simulink library "SUB_ECU_L4_MABX"  (R2018a)
settings: Solver=VariableStepAuto  StartTime=0.0  StopTime=10.0  RelTol=1e-3
libraries: EmE_MBD_Blockset x76, simulink x14, SUB_L4_Task_10000ms x1, SUB_L4_Task_1000ms x1, SUB_L4_Task_100ms x1, SUB_L4_Task_10ms_SUB_APTC x1, PTC_MBDS_LIB x1, SUB_L4_Task_10ms_SUB_BRKPEDARB x1, SUB_L4_Task_10ms_SUB_FAULT_MANAGER x1, SUB_L4_Task_10ms_SUB_STATE_CONTROL x1, SUB_L4_Task_10ms_SUB_STEERCTRL x1, simulink_need_slupdate x1
(part 2 of 2)

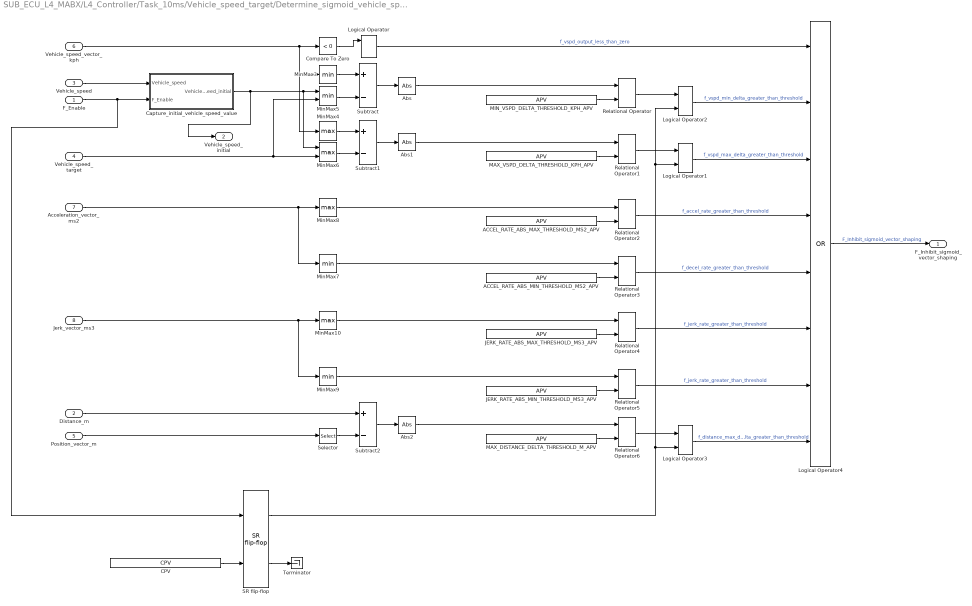
== system SUB_ECU_L4_MABX/L4_Controller/Task_10ms/Vehicle_speed_target/Determine_sigmoid_vehicle_speed_profile/Determine_inhibit_sigmoid_vehicle_speed_profile ==
  F_Enable : Inport
  Distance_m : Inport  Port=2
  Vehicle_speed : Inport  Port=3
  Vehicle_speed_target : Inport  Port=4
  Position_vector_m : Inport  Port=5
  Vehicle_speed_vector_kph : Inport  Port=6
  Acceleration_vector_ms2 : Inport  Port=7
  Jerk_vector_ms3 : Inport  Port=8
  ACCEL_RATE_ABS_MAX_THRESHOLD_MS2_APV : EmE_MBD_Blockset/Sources/APV  conval=5
      settings: SourceProductName=PACCAR EmE MBD Blockset
  ACCEL_RATE_ABS_MIN_THRESHOLD_MS2_APV : EmE_MBD_Blockset/Sources/APV  conval=-5
      settings: SourceProductName=PACCAR EmE MBD Blockset
  Abs : EmE_MBD_Blockset/Math Operators/Abs
      settings: SourceProductName=PACCAR EmE MBD Blockset
  Abs1 : EmE_MBD_Blockset/Math Operators/Abs
      settings: SourceProductName=PACCAR EmE MBD Blockset
  Abs2 : EmE_MBD_Blockset/Math Operators/Abs
      settings: SourceProductName=PACCAR EmE MBD Blockset
  CPV : EmE_MBD_Blockset/Sources/CPV  conval=false
      settings: SourceProductName=PACCAR EmE MBD Blockset
  Capture_initial_vehicle_speed_value : Subsystem
  Compare To Zero : simulink/Logic and Bit Operations/Compare To Zero  relop=<  OutDataTypeStr=boolean
  JERK_RATE_ABS_MAX_THRESHOLD_MS3_APV : EmE_MBD_Blockset/Sources/APV  conval=5
      settings: SourceProductName=PACCAR EmE MBD Blockset
  JERK_RATE_ABS_MIN_THRESHOLD_MS3_APV : EmE_MBD_Blockset/Sources/APV  conval=-5
      settings: SourceProductName=PACCAR EmE MBD Blockset
  Logical Operator : EmE_MBD_Blockset/Logic and Bit Operations/Logical Operator  Operator=OR  Inputs=1
      settings: SourceProductName=PACCAR EmE MBD Blockset
  Logical Operator1 : EmE_MBD_Blockset/Logic and Bit Operations/Logical Operator  Operator=AND  Inputs=2
      settings: SourceProductName=PACCAR EmE MBD Blockset
  Logical Operator2 : EmE_MBD_Blockset/Logic and Bit Operations/Logical Operator  Operator=AND  Inputs=2
      settings: SourceProductName=PACCAR EmE MBD Blockset
  Logical Operator3 : EmE_MBD_Blockset/Logic and Bit Operations/Logical Operator  Operator=AND  Inputs=2
      settings: SourceProductName=PACCAR EmE MBD Blockset
  Logical Operator4 : Logic  Operator=OR  Inputs=8  AllPortsSameDT=off  OutDataTypeStr=boolean
  MAX_DISTANCE_DELTA_THRESHOLD_M_APV : EmE_MBD_Blockset/Sources/APV  conval=0.5
      settings: SourceProductName=PACCAR EmE MBD Blockset
  MAX_VSPD_DELTA_THRESHOLD_KPH_APV : EmE_MBD_Blockset/Sources/APV  conval=5
      settings: SourceProductName=PACCAR EmE MBD Blockset
  MIN_VSPD_DELTA_THRESHOLD_KPH_APV : EmE_MBD_Blockset/Sources/APV  conval=5
      settings: SourceProductName=PACCAR EmE MBD Blockset
  MinMax10 : MinMax  Function=max  InputSameDT=on
  MinMax3 : MinMax  InputSameDT=on
  MinMax4 : MinMax  Function=max  InputSameDT=on
  MinMax5 : MinMax  Inputs=2  InputSameDT=on
  MinMax6 : MinMax  Function=max  Inputs=2  InputSameDT=on
  MinMax7 : MinMax  InputSameDT=on
  MinMax8 : MinMax  Function=max  InputSameDT=on
  MinMax9 : MinMax  InputSameDT=on
  Relational Operator{,1..2,4,6} (5 alike) : EmE_MBD_Blockset/Logic and Bit Operations/Relational Operator  func=>
      settings: SourceProductName=PACCAR EmE MBD Blockset
  Relational Operator3 : EmE_MBD_Blockset/Logic and Bit Operations/Relational Operator  func=<
      settings: SourceProductName=PACCAR EmE MBD Blockset
  Relational Operator5 : EmE_MBD_Blockset/Logic and Bit Operations/Relational Operator  func=<
      settings: SourceProductName=PACCAR EmE MBD Blockset
  SR flip-flop : EmE_MBD_Blockset/Logic and Bit Operations/SR flip-flop
      settings: SourceProductName=PACCAR EmE MBD Blockset
  Selector : Selector  InputPortWidth=33  IndexOptions=Index vector (dialog)  Indices=33  OutputSizes=1
  Subtract : Sum  Inputs=+-  InputSameDT=on
  Subtract1 : Sum  Inputs=+-  InputSameDT=on
  Subtract2 : Sum  Inputs=+-  InputSameDT=on
  Terminator : Terminator
  F_Inhibit_sigmoid_vector_shaping : Outport  LibraryBlock=EmE_MBD_Blockset/Sinks/Out  OutputWhenDisabled=reset
  Vehicle_speed_initial : Outport  Port=2
  wires:
  Relational Operator6/1 -> Logical Operator3/1
  Position_vector_m/1 -> Selector/1
  Selector/1 -> Subtract2/2
  Logical Operator3/1 -> Logical Operator4/8  "f_distance_max_delta_greater_than_threshold"
  Distance_m/1 -> Subtract2/1
  Subtract2/1 -> Abs2/1
  Abs2/1 -> Relational Operator6/1
  MAX_DISTANCE_DELTA_THRESHOLD_M_APV/1 -> Relational Operator6/2
  Vehicle_speed/1 -> Capture_initial_vehicle_speed_value/1(Vehicle_speed)
  Capture_initial_vehicle_speed_value/1(Vehicle_speed_initial) -> MinMax5/1, MinMax6/1, Vehicle_speed_initial/1
  Vehicle_speed_target/1 -> MinMax6/2, MinMax5/2
  MinMax6/1 -> Subtract1/2
  MinMax5/1 -> Subtract/2
  Subtract/1 -> Abs/1
  Subtract1/1 -> Abs1/1
  Relational Operator1/1 -> Logical Operator1/1
  MAX_VSPD_DELTA_THRESHOLD_KPH_APV/1 -> Relational Operator1/2
  Logical Operator2/1 -> Logical Operator4/2  "f_vspd_min_delta_greater_than_threshold"
  MinMax9/1 -> Relational Operator5/1
  JERK_RATE_ABS_MIN_THRESHOLD_MS3_APV/1 -> Relational Operator5/2
  Logical Operator/1 -> Logical Operator4/1  "f_vspd_output_less_than_zero"
  MinMax4/1 -> Subtract1/1
  MIN_VSPD_DELTA_THRESHOLD_KPH_APV/1 -> Relational Operator/2
  Jerk_vector_ms3/1 -> MinMax10/1, MinMax9/1
  Abs1/1 -> Relational Operator1/1
  Abs/1 -> Relational Operator/1
  Logical Operator1/1 -> Logical Operator4/3  "f_vspd_max_delta_greater_than_threshold"
  Relational Operator5/1 -> Logical Operator4/7  "f_jerk_rate_greater_than_threshold"
  MinMax10/1 -> Relational Operator4/1
  ACCEL_RATE_ABS_MAX_THRESHOLD_MS2_APV/1 -> Relational Operator2/2
  MinMax8/1 -> Relational Operator2/1
  Relational Operator/1 -> Logical Operator2/1
  JERK_RATE_ABS_MAX_THRESHOLD_MS3_APV/1 -> Relational Operator4/2
  Acceleration_vector_ms2/1 -> MinMax8/1, MinMax7/1
  Vehicle_speed_vector_kph/1 -> Compare To Zero/1, MinMax3/1, MinMax4/1
  Relational Operator2/1 -> Logical Operator4/4  "f_accel_rate_greater_than_threshold"
  Relational Operator3/1 -> Logical Operator4/5  "f_decel_rate_greater_than_threshold"
  MinMax3/1 -> Subtract/1
  SR flip-flop/1 -> Logical Operator2/2, Logical Operator1/2, Logical Operator3/2
  MinMax7/1 -> Relational Operator3/1
  SR flip-flop/2 -> Terminator/1
  Relational Operator4/1 -> Logical Operator4/6  "f_jerk_rate_greater_than_threshold"
  CPV/1 -> SR flip-flop/2
  Logical Operator4/1 -> F_Inhibit_sigmoid_vector_shaping/1  "F_Inhibit_sigmoid_vector_shaping"
  ACCEL_RATE_ABS_MIN_THRESHOLD_MS2_APV/1 -> Relational Operator3/2
  F_Enable/1 -> Capture_initial_vehicle_speed_value/2(F_Enable), SR flip-flop/1
  Compare To Zero/1 -> Logical Operator/1

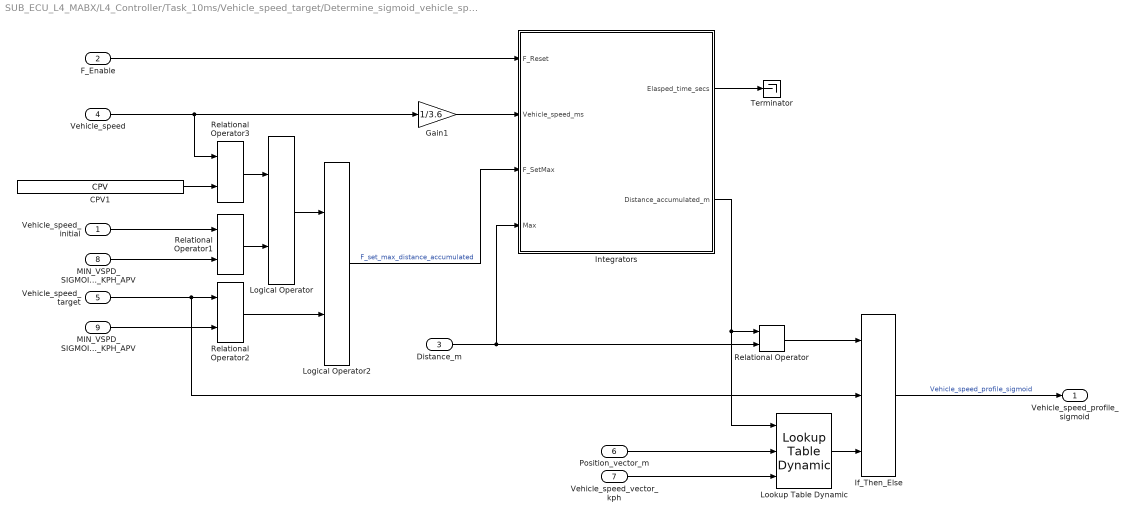
== system SUB_ECU_L4_MABX/L4_Controller/Task_10ms/Vehicle_speed_target/Determine_sigmoid_vehicle_speed_profile/Select_vehicle_speed_target_value ==
  Vehicle_speed_initial : Inport
  F_Enable : Inport  Port=2
  Distance_m : Inport  Port=3
  Vehicle_speed : Inport  Port=4
  Vehicle_speed_target : Inport  Port=5
  Position_vector_m : Inport  Port=6
  Vehicle_speed_vector_kph : Inport  Port=7
  MIN_VSPD_SIGMOID_INITIAL_KPH_APV : Inport  Port=8
  MIN_VSPD_SIGMOID_FINAL_KPH_APV : Inport  Port=9
  CPV1 : EmE_MBD_Blockset/Sources/CPV  conval=0.1
      settings: SourceProductName=PACCAR EmE MBD Blockset
  Gain1 : Gain  Gain=1/3.6
  If_Then_Else : EmE_MBD_Blockset/Signal Routing/If_Then_Else
      settings: SourceProductName=PACCAR EmE MBD Blockset
  Integrators : Subsystem
  Logical Operator : EmE_MBD_Blockset/Logic and Bit Operations/Logical Operator  Operator=OR  Inputs=2
      settings: SourceProductName=PACCAR EmE MBD Blockset
  Logical Operator2 : EmE_MBD_Blockset/Logic and Bit Operations/Logical Operator  Operator=AND  Inputs=2
      settings: SourceProductName=PACCAR EmE MBD Blockset
  Lookup Table Dynamic : simulink/Lookup Tables/Lookup Table Dynamic  LookUpMeth=Interpolation-Use End Values  OutDataType=fixdt('double')  OutScaling=[]  OutputDataTypeScalingMode=Specify via dialog  OutDataTypeStr=double  DoSatur=off
      settings: SourceProductName=Simulink
  Relational Operator : EmE_MBD_Blockset/Logic and Bit Operations/Relational Operator  func===
      settings: SourceProductName=PACCAR EmE MBD Blockset
  Relational Operator1 : EmE_MBD_Blockset/Logic and Bit Operations/Relational Operator  func=<
      settings: SourceProductName=PACCAR EmE MBD Blockset
  Relational Operator2 : EmE_MBD_Blockset/Logic and Bit Operations/Relational Operator  func=<
      settings: SourceProductName=PACCAR EmE MBD Blockset
  Relational Operator3 : EmE_MBD_Blockset/Logic and Bit Operations/Relational Operator  func=<
      settings: SourceProductName=PACCAR EmE MBD Blockset
  Terminator : Terminator
  Vehicle_speed_profile_sigmoid : Outport
  wires:
  Logical Operator2/1 -> Integrators/3(F_SetMax)  "F_set_max_distance_accumulated"
  CPV1/1 -> Relational Operator3/2
  Relational Operator1/1 -> Logical Operator/2
  Logical Operator/1 -> Logical Operator2/1
  Relational Operator3/1 -> Logical Operator/1
  Relational Operator/1 -> If_Then_Else/1
  Gain1/1 -> Integrators/2(Vehicle_speed_ms)
  Integrators/2(Distance_accumulated_m) -> Relational Operator/1, Lookup Table Dynamic/1
  MIN_VSPD_SIGMOID_FINAL_KPH_APV/1 -> Relational Operator2/2
  MIN_VSPD_SIGMOID_INITIAL_KPH_APV/1 -> Relational Operator1/2
  Relational Operator2/1 -> Logical Operator2/2
  Vehicle_speed_initial/1 -> Relational Operator1/1
  F_Enable/1 -> Integrators/1(F_Reset)
  Lookup Table Dynamic/1 -> If_Then_Else/3
  Vehicle_speed_vector_kph/1 -> Lookup Table Dynamic/3
  Integrators/1(Elasped_time_secs) -> Terminator/1
  Position_vector_m/1 -> Lookup Table Dynamic/2
  Vehicle_speed/1 -> Gain1/1, Relational Operator3/1
  Distance_m/1 -> Integrators/4(Max), Relational Operator/2
  If_Then_Else/1 -> Vehicle_speed_profile_sigmoid/1  "Vehicle_speed_profile_sigmoid"
  Vehicle_speed_target/1 -> Relational Operator2/1, If_Then_Else/2

== system SUB_ECU_L4_MABX/L4_Controller/Task_10ms/Vehicle_speed_target/Determine_sigmoid_vehicle_speed_profile/Determine_inhibit_sigmoid_vehicle_speed_profile/Capture_initial_vehicle_speed_value ==
  Vehicle_speed : Inport
  F_Enable : Inport  Port=2
  If_Then_Else : EmE_MBD_Blockset/Signal Routing/If_Then_Else
      settings: SourceProductName=PACCAR EmE MBD Blockset
  Unit_Delay : UnitDelay  SampleTime=-1
      settings: AttributesFormatString=IC: %<vinit>
  Vehicle_speed_initial : Outport
  wires:
  Vehicle_speed/1 -> If_Then_Else/2
  Unit_Delay/1 -> If_Then_Else/3
  F_Enable/1 -> If_Then_Else/1
  If_Then_Else/1 -> Vehicle_speed_initial/1, Unit_Delay/1  "Vehicle_speed_initial"

== system SUB_ECU_L4_MABX/L4_Controller/Task_10ms/Vehicle_speed_target/Determine_sigmoid_vehicle_speed_profile/Select_vehicle_speed_target_value/Integrators ==
  F_Reset : Inport
  Vehicle_speed_ms : Inport  Port=2
  F_SetMax : Inport  Port=3
  Max : Inport  Port=4
  CPV : EmE_MBD_Blockset/Sources/CPV  conval=1
      settings: SourceProductName=PACCAR EmE MBD Blockset
  CPV1 : EmE_MBD_Blockset/Sources/CPV  conval=1
      settings: SourceProductName=PACCAR EmE MBD Blockset
  CPV2 : EmE_MBD_Blockset/Sources/CPV  conval=1
      settings: SourceProductName=PACCAR EmE MBD Blockset
  CalculateDistance : Subsystem
  Discrete-Time Integrator : EmE_MBD_Blockset/Discrete/Discrete-Time Integrator  integrator_method_sel=Backward Euler
      settings: AttributesFormatString=%<integrator_method_sel>  SourceProductName=PACCAR EmE MBD Blockset
  dT : EmE_MBD_Blockset/Sources/dT
      settings: SourceProductName=PACCAR EmE MBD Blockset
  dT1 : EmE_MBD_Blockset/Sources/dT
      settings: SourceProductName=PACCAR EmE MBD Blockset
  Elasped_time_secs : Outport
  Distance_accumulated_m : Outport  Port=2
  wires:
  F_SetMax/1 -> CalculateDistance/5(F_SetMax)
  Max/1 -> CalculateDistance/6(Max)
  CPV2/1 -> Discrete-Time Integrator/2
  CPV1/1 -> CalculateDistance/3(K)
  dT1/1 -> CalculateDistance/4(dT)
  Discrete-Time Integrator/1 -> Elasped_time_secs/1  "Elasped_time_secs"
  F_Reset/1 -> Discrete-Time Integrator/1, CalculateDistance/1(F_Reset)
  Vehicle_speed_ms/1 -> CalculateDistance/2(U)
  CPV/1 -> Discrete-Time Integrator/3
  CalculateDistance/1(Y) -> Distance_accumulated_m/1  "Distance_accumulated_m"
  dT/1 -> Discrete-Time Integrator/4

== system SUB_ECU_L4_MABX/L4_Controller/Task_10ms/Vehicle_speed_target/Determine_sigmoid_vehicle_speed_profile/Select_vehicle_speed_target_value/Integrators/CalculateDistance ==
  F_Reset : Inport
  U : Inport  Port=2
  K : Inport  Port=3
  dT : Inport  Port=4
  F_SetMax : Inport  Port=5
  Max : Inport  Port=6
  Add : Sum  InputSameDT=on
  CPV : EmE_MBD_Blockset/Sources/CPV  conval=0
      settings: SourceProductName=PACCAR EmE MBD Blockset
  If_Then_Else : EmE_MBD_Blockset/Signal Routing/If_Then_Else
      settings: SourceProductName=PACCAR EmE MBD Blockset
  MinMax : MinMax  Inputs=2  InputSameDT=on
  Product1 : Product  Inputs=3  InputSameDT=on
  Unit Delay Resettable External IC1 : simulink_need_slupdate/Unit Delay Resettable External IC  tsamp=-1
      settings: SourceProductName=Simulink  SourceProductBaseCode=SL
  Y : Outport  OutputWhenDisabled=reset  InitialOutput=0
  wires:
  F_Reset/1 -> Unit Delay Resettable External IC1/2
  Product1/1 -> Add/2
  Add/1 -> MinMax/2
  CPV/1 -> Unit Delay Resettable External IC1/3
  Unit Delay Resettable External IC1/1 -> Add/1
  If_Then_Else/1 -> Y/1, Unit Delay Resettable External IC1/1
  MinMax/1 -> If_Then_Else/3
  F_SetMax/1 -> If_Then_Else/1
  Max/1 -> If_Then_Else/2, MinMax/1
  dT/1 -> Product1/3
  K/1 -> Product1/1
  U/1 -> Product1/2

== stateflow chart SUB_ECU_L4_MABX/L4_Controller/Task_10ms/Vehicle_speed_target/Determine_sigmoid_vehicle_speed_profile/TwentyPointVectorCalculation ==
  (default) -> (junction 85)
  (junction 85) -> (junction 86) [order 1] : [Enable]
  (junction 85) -> (junction 87) [order 2]
  (junction 86) -> (junction 21) : {TimeVector(1) = TimeVectorRaw(1);
      | JerkVector(1) = JerkVectorRaw(1);
      | AccelerationVector(1) = AccelerationVectorRaw(1);
      | VelocityVector(1) = VelocityVectorRaw(1);
      | PositionVector(1) = PositionVectorRaw(1);
      |
      | TimeIncrement = (TimeVectorRaw(2) - TimeVectorRaw(1)) / 10;
      | i = 2;}
  (junction 21) -> (junction 19) [order 1] : [i <= 10]
  (junction 19) -> (junction 22) : {TimeVector(i) = TimeVector(i-1) + TimeIncrement;
      | DeltaTime = TimeVector(i) - TimeVectorRaw(1);
      | JerkVector(i) = JerkVectorRaw(1);
      | AccelerationVector(i) = AccelerationVectorRaw(1) + JerkVectorRaw(1) * DeltaTime;
      | VelocityVector(i) = VelocityVectorRaw(1) + AccelerationVectorRaw(1) * DeltaTime + 0.5 * JerkVectorRaw(1) * DeltaTime^2;
      | PositionVector(i) = PositionVectorRaw(1) + VelocityVectorRaw(1) * DeltaTime + 0.5 * AccelerationVectorRaw(1) * DeltaTime^2 + (JerkVectorRaw(1) / 6) * DeltaTime^3;
      | PositionVector(i) = max(PositionVector(i-1) + 0.0001, PositionVector(i));}
  (junction 22) -> (junction 21) : {i = i + 1;}
  (junction 21) -> (junction 129) [order 2] : {TimeVector(11) = TimeVectorRaw(2);
      | JerkVector(11) = JerkVectorRaw(2);
      | AccelerationVector(11) = AccelerationVectorRaw(2);
      | VelocityVector(11) = VelocityVectorRaw(2);
      | PositionVector(11) = max(PositionVector(10) + 0.0001, PositionVectorRaw(2));
      |
      | TimeVector(12) = TimeVectorRaw(3);
      | JerkVector(12) = JerkVectorRaw(3);
      | AccelerationVector(12) = AccelerationVectorRaw(3);
      | VelocityVector(12) = VelocityVectorRaw(3);
      | PositionVector(12) = max(PositionVector(11) + 0.0001, PositionVectorRaw(3));
      |
      | TimeIncrement = (TimeVectorRaw(4) - TimeVectorRaw(3)) / 10;
      | i = 13;}
  (junction 129) -> (junction 128) [order 1] : [i <= 21]
  (junction 128) -> (junction 130) : {TimeVector(i) = TimeVector(i-1) + TimeIncrement;
      | DeltaTime = TimeVector(i) - TimeVectorRaw(3);
      | JerkVector(i) = JerkVectorRaw(3);
      | AccelerationVector(i) = AccelerationVectorRaw(3) + JerkVectorRaw(3) * DeltaTime;
      | VelocityVector(i) = VelocityVectorRaw(3) + AccelerationVectorRaw(3) * DeltaTime + 0.5 * JerkVectorRaw(3) * DeltaTime^2;
      | PositionVector(i) = PositionVectorRaw(3) + VelocityVectorRaw(3) * DeltaTime + 0.5 * AccelerationVectorRaw(3) * DeltaTime^2 + (JerkVectorRaw(3) / 6) * DeltaTime^3;
      | PositionVector(i) = max(PositionVector(i-1) + 0.0001, PositionVector(i));}
  (junction 130) -> (junction 129) : {i = i + 1;}
  (junction 129) -> (junction 109) [order 2] : {TimeVector(22) = TimeVectorRaw(4);
      | JerkVector(22) = JerkVectorRaw(4);
      | AccelerationVector(22) = AccelerationVectorRaw(4);
      | VelocityVector(22) = VelocityVectorRaw(4);
      | PositionVector(22) = max(PositionVector(21) + 0.0001, PositionVectorRaw(4));
      |
      | TimeVector(23) = TimeVectorRaw(5);
      | JerkVector(23) = JerkVectorRaw(5);
      | AccelerationVector(23) = AccelerationVectorRaw(5);
      | VelocityVector(23) = VelocityVectorRaw(5);
      | PositionVector(23) = max(PositionVector(22) + 0.0001, PositionVectorRaw(5));
      |
      | TimeIncrement = (TimeVectorRaw(6) - TimeVectorRaw(5)) / 10;
      | i = 24;}
  (junction 109) -> (junction 107) [order 1] : [i <= 32]
  (junction 107) -> (junction 108) : {TimeVector(i) = TimeVector(i-1) + TimeIncrement;
      | DeltaTime = TimeVector(i) - TimeVectorRaw(5);
      | JerkVector(i) = JerkVectorRaw(5);
      | AccelerationVector(i) = AccelerationVectorRaw(5) + JerkVectorRaw(5) * DeltaTime;
      | VelocityVector(i) = VelocityVectorRaw(5) + AccelerationVectorRaw(5) * DeltaTime + 0.5 * JerkVectorRaw(5) * DeltaTime^2;
      | PositionVector(i) = PositionVectorRaw(5) + VelocityVectorRaw(5) * DeltaTime + 0.5 * AccelerationVectorRaw(5) * DeltaTime^2 + (JerkVectorRaw(5) / 6) * DeltaTime^3;
      | PositionVector(i) = max(PositionVector(i-1) + 0.0001, PositionVector(i));}
  (junction 108) -> (junction 109) : {i = i + 1;}
  (junction 109) -> (junction 23) [order 2] : {TimeVector(33) = TimeVectorRaw(6);
      | JerkVector(33) = JerkVectorRaw(6);
      | AccelerationVector(33) = AccelerationVectorRaw(6);
      | VelocityVector(33) = VelocityVectorRaw(6);
      | PositionVector(33) = max(PositionVector(32) + 0.0001, PositionVectorRaw(6));}
  (junction 23) -> (junction 87)
  (junction 87) -> (junction 92)
  data: TimeVector output size=33 =[0:0.001:0.032]'; PositionVector output size=33 =[0:0.001:0.032]'; VelocityVector output size=33 =zeros(33,1); AccelerationVector output size=33 =zeros(33,1); JerkVector output size=33 =zeros(33,1); Enable input; PositionFinal input; TimeVectorRaw input; PositionVectorRaw input; VelocityVectorRaw input; AccelerationVectorRaw input; JerkVectorRaw input; i local uint8; DeltaTime local double; TimeIncrement local double

== stateflow chart SUB_ECU_L4_MABX/L4_Controller/Task_10ms/Vehicle_speed_target/Determine_sigmoid_vehicle_speed_profile/VehicleSpeedSetpointDynamicCalculation ==
  state CalculateAcceleration34 [function]
    (default) -> (junction 180) : {num = 2 * (AccelerationInitialLimited *  AccelerationFinalLimited ...
        |     - AccelerationInitialLimited * Jerk56 * TimeFinal ...
        |     + Jerk56 * (VelocityFinalLimited - VelocityInitialLimited)) ...
        |     - AccelerationInitialLimited^2 - AccelerationFinalLimited^2;
        |
        | den = 2 * ((VelocityFinalLimited - VelocityInitialLimited) ...
        |     - AccelerationFinalLimited * TimeFinal) ...
        |     + Jerk56 * TimeFinal^2;
        |
        | Jerk12 = sign(Jerk12) * max(abs(Jerk12), abs(num / den) + 0.001);
        | Jerk12 = max(-10,min(10,Jerk12));
        |
        | Calculate_abc}
    (junction 180) -> (junction 181) [order 1] : [abs(a) < 0.01 ]
    (junction 180) -> (junction 205) [order 2]
    (junction 181) -> (junction 183) : {Jerk12 = Jerk56;
        | Calculate_abc
        | Acceleration34 = - c / b;
        | AlternateMethod = false;}
    (junction 205) -> (junction 291) [order 1] : [b^2 <= 4 * a * c]
    (junction 205) -> (junction 288) [order 2] : {Acceleration34 = (- b + (b^2 - 4 * a * c)^0.5) / (2 * a);
        | AlternateMethod = false;}
    (junction 291) -> (junction 290) : {CalculateAlternate_abc
        | Acceleration34 = - b / (2 * a);
        | AlternateMethod = true;}
    (junction 290) -> (junction 288)
    (junction 183) -> (junction 290)
    (junction 288) -> (junction 189)
  state Calculate_abc [function]
    (default) -> (junction 164) : {a = Jerk56 - Jerk12;
        | b = 2 * (AccelerationFinalLimited * Jerk12 - AccelerationInitialLimited * Jerk56 - Jerk12 * Jerk56 * TimeFinal);
        | c = 2 * Jerk12 * Jerk56 * (VelocityFinalLimited - VelocityInitialLimited) + Jerk56 * AccelerationInitialLimited^2 - Jerk12 * AccelerationFinalLimited^2;}
  state CalculateAlternate_abc [function]
    (default) -> (junction 287) : {a = 1;
        | b = 2 * (Jerk56 * (TimeFinal - 0.005) - AccelerationFinalLimited);
        | c = 2 * Jerk56 * (VelocityInitialLimited - VelocityFinalLimited) + AccelerationFinalLimited^2;}
  (default) -> (junction 85)
  (junction 85) -> (junction 86) [order 1] : [Enable]
  (junction 85) -> (junction 87) [order 2]
  (junction 86) -> (junction 236) : {PositionFinalLimited = max(0.001,PositionFinal);  % limit minimum distance so that values in PositionVectorRaw are in increasing order
      |
      | VelocityInitialLimited = max(0.1,VelocityInitial);  % limit to make sure FinalTime calculation does not divide by zero
      | VelocityFinalLimited = max(0.1,VelocityFinal);  % limit to make sure FinalTime calculation does not divide by zero
      |
      | TimeFinal = 2 * PositionFinalLimited / (VelocityInitialLimited + VelocityFinalLimited);  % first approximation for total time
      | TimeFinal = max(0.007, TimeFinal);  % limit to make sure values in JerkVectorRaw are in increasing order and divide by zero protection
      |  AccelerationAverage = (VelocityFinalLimited - VelocityInitialLimited) / TimeFinal;   % acceleration with straight line velocity change
      | TimeFinal = 2 * TimeFinal;  % increase initial estimate two times to make sure solution is within search range
      | }
  (junction 236) -> (junction 237) [order 1] : [VelocityFinalLimited > VelocityInitialLimited]
  (junction 236) -> (junction 38) [order 2] : {% deceleration sigmoid limits
      | AccelerationInitialLimited = max(AccelerationAverage, min(0, AccelerationInitial));
      | AccelerationFinalLimited = max(AccelerationAverage, min(0, AccelerationFinal));}
  (junction 237) -> (junction 239) : {% acceleration sigmoid limits
      | AccelerationInitialLimited = max(0, min(AccelerationAverage, AccelerationInitial));
      | AccelerationFinalLimited = max(0, min(AccelerationAverage, AccelerationFinal));}
  (junction 239) -> (junction 38)
  (junction 38) -> (junction 21) : {DeltaTimeFinal = TimeFinal;  % initialize DeltaTimeFinal term for binary search
      | i = 1;}
  (junction 21) -> (junction 19) [order 1] : % TimeFinal
      | % Binary Search
      |
      | [i <= 15]
  (junction 19) -> (junction 115) : {JerkFinalMinimum = 2 * (VelocityInitialLimited - VelocityFinalLimited + AccelerationFinalLimited * TimeFinal) / TimeFinal^2;}
  (junction 115) -> (junction 117) [order 1] : [VelocityFinalLimited > VelocityInitialLimited]
  (junction 115) -> (junction 269) [order 2] : {% deceleration
      | Jerk12 = -JerkMagnitudeInitial;
      | Jerk56 = max(abs(JerkFinalMinimum), JerkMagnitudeFinal);}
  (junction 117) -> (junction 119) : {% acceleration
      | Jerk12 = JerkMagnitudeInitial;
      | Jerk56 = -max(abs(JerkFinalMinimum), JerkMagnitudeFinal);}
  (junction 119) -> (junction 269)
  (junction 269) -> (junction 25) : {CalculateAcceleration34}
  (junction 25) -> (junction 143) [order 1] : [abs(Acceleration34 - AccelerationAverage) < 0.001]
  (junction 25) -> (junction 297) [order 2]
  (junction 143) -> (junction 149) : {Time12 = 0.002;
      | Time56 = 0.002;
      |
      | TimeVectorRaw = [0; Time12 - 0.001; Time12 + 0.001; ...
      |     TimeFinal - Time56 - 0.001; TimeFinal - Time56 + 0.001;TimeFinal];
      |
      | JerkVectorRaw = [0; 0; 0; 0; 0; 0];
      | AccelerationVectorRaw(1) = AccelerationAverage;}
  (junction 297) -> (junction 299) [order 1] : [AlternateMethod]
  (junction 297) -> (junction 156) [order 2] : {Time12 = max(0.002, (Acceleration34 - AccelerationInitialLimited) / Jerk12);
      | Time56 = max(0.002, (AccelerationFinalLimited - Acceleration34) / Jerk56);
      |
      | TimeVectorRaw = [0; Time12 - 0.001; Time12 + 0.001; ...
      |     TimeFinal - Time56 - 0.001; TimeFinal - Time56 + 0.001;TimeFinal];
      |
      | JerkVectorRaw = [Jerk12; Jerk12; 0; 0; Jerk56; Jerk56];
      | AccelerationVectorRaw(1) = AccelerationInitialLimited;}
  (junction 299) -> (junction 301) : {Time12 = 0.002;
      | Time56 = max(0.002, (AccelerationFinalLimited - Acceleration34) / Jerk56);
      |
      | TimeVectorRaw = [0; Time12 - 0.001; Time12 + 0.001; ...
      |     TimeFinal - Time56 - 0.001; TimeFinal - Time56 + 0.001;TimeFinal];
      |
      | JerkVectorRaw = [0; 0; 0; 0; Jerk56; Jerk56];
      | AccelerationVectorRaw(1) = Acceleration34;}
  (junction 301) -> (junction 156)
  (junction 149) -> (junction 301)
  (junction 22) -> (junction 21) : {i = i + 1;}
  (junction 21) -> (junction 23) [order 2]
  (junction 156) -> (junction 32) : {VelocityVectorRaw(1) = VelocityInitialLimited;
      | PositionVectorRaw(1) = 0;
      | j = 2;}
  (junction 32) -> (junction 35) [order 1] : [j <= 6]
  (junction 35) -> (junction 31) : {DeltaTime = TimeVectorRaw(j) - TimeVectorRaw(j-1);
      | AverageJerk = 0.5 * (JerkVectorRaw(j-1) + JerkVectorRaw(j));
      | AccelerationVectorRaw(j) = AccelerationVectorRaw(j-1) + JerkVectorRaw(j-1) * DeltaTime;
      | VelocityVectorRaw(j) = VelocityVectorRaw(j-1) + AccelerationVectorRaw(j-1) * DeltaTime + 0.5 * JerkVectorRaw(j-1) * DeltaTime^2;
      | PositionVectorRaw(j) = PositionVectorRaw(j-1) + VelocityVectorRaw(j-1) * DeltaTime + 0.5 * AccelerationVectorRaw(j-1) * DeltaTime^2 + (JerkVectorRaw(j-1) / 6) * DeltaTime^3;}
  (junction 31) -> (junction 32) : {j = j + 1;}
  (junction 32) -> (junction 56) [order 2] : {PositionError = PositionVectorRaw(end) - PositionFinalLimited;
      | DeltaTimeFinal = 0.5 * DeltaTimeFinal;  % reduce DeltaTimeFinal by 50 percent on each iteration of the search
      | }
  (junction 56) -> (junction 57) [order 1] : [(PositionError < 0) && (VelocityVectorRaw(end) > 0)]
  (junction 56) -> (junction 59) [order 2] : {TimeFinal = TimeFinal - DeltaTimeFinal;}
  (junction 57) -> (junction 58) : {TimeFinal = TimeFinal + DeltaTimeFinal;}
  (junction 58) -> (junction 59)
  (junction 59) -> (junction 22) : {TimeFinal = max(0.007, TimeFinal);}
  (junction 23) -> (junction 87)
  (junction 87) -> (junction 92)
  data: TimeVectorRaw output size=6 =[0:0.001:0.005]'; PositionVectorRaw output size=6 =[0:0.001:0.005]'; VelocityVectorRaw output size=6 =zeros(6,1); AccelerationVectorRaw output size=6 =zeros(6,1); JerkVectorRaw output size=6 =zeros(6,1); Enable input boolean; PositionFinal input; VelocityInitial input; VelocityFinal input; AccelerationInitial input; AccelerationFinal input; TimeFinal local double; AccelerationAverage local double; DeltaTimeFinal local double; i local uint8; j local uint8; DeltaTime local double; AverageJerk local double; PositionError local double; JerkError local double; PositionFinalLimited local double; VelocityInitialLimited local double; VelocityFinalLimited local double; AccelerationInitialLimited local double; AccelerationFinalLimited local double; Jerk56 local double; Jerk12 local double; JerkMagnitudeInitial input; JerkMagnitudeFinal input; a local double; b local double; c local double; Acceleration34 local double; Time12 local double; Time56 local double; JerkFinalMinimum local double; AlternateMethod local boolean; num local double; den local double
